simulink model "practica09"  (R2024a)
settings: Solver=VariableStepAuto  StartTime=0.0  StopTime=15  RelTol=1e-3
libraries: simulink_extras x1

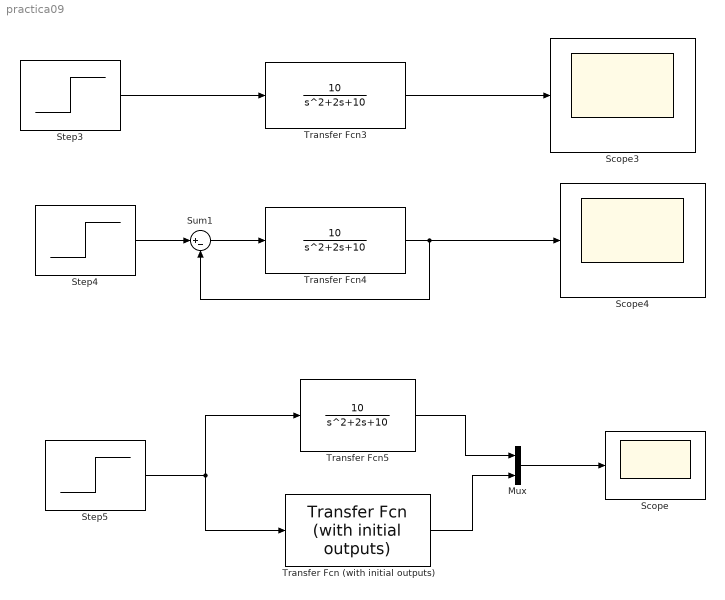
== system practica09 ==
  Mux : Mux  Inputs=2
  Scope : Scope
  Scope3 : Scope
  Scope4 : Scope
  Step3 : Step  Time=0  After=2  SampleTime=0
  Step4 : Step  Time=0  After=2  SampleTime=0
  Step5 : Step  Time=0  After=2  SampleTime=0
  Sum1 : Sum  Inputs=|+-
  Transfer Fcn (with initial outputs) : simulink_extras/Additional Linear/Transfer Fcn (with initial outputs)  N=[1 0]  D="[1  5]"  Y0=.5  U0=0
  Transfer Fcn3 : TransferFcn  Numerator=[10]  Denominator=[1 2 10]
  Transfer Fcn4 : TransferFcn  Numerator=[10]  Denominator=[1 2 10]
  Transfer Fcn5 : TransferFcn  Numerator=[10]  Denominator=[1 2 10]
  wires:
  Sum1/1 -> Transfer Fcn4/1
  Step4/1 -> Sum1/1
  Transfer Fcn3/1 -> Scope3/1
  Transfer Fcn4/1 -> Scope4/1, Sum1/2
  Step3/1 -> Transfer Fcn3/1
  Step5/1 -> Transfer Fcn5/1, Transfer Fcn (with initial outputs)/1
  Transfer Fcn5/1 -> Mux/1
  Transfer Fcn (with initial outputs)/1 -> Mux/2
  Mux/1 -> Scope/1
